simulink model "newsldrt2018"  (R2018b)
settings: Solver=ode5  StartTime=0.0  StopTime=10  FixedStep=1  RelTol=1e-3  EnableMultiTasking=on
model workspace (MAT data in the model file):
  A = 20
  a = 2
  b = 5
libraries: simulink x1
settings Model: Creator=The MathWorks, Inc.  LastModifiedBy=hp
settings SolverCC: ConcurrentTasks=on  PositivePriorityOrder=on
settings DataIOCC: ExternalInput=getinputstruct(op_watertank_comp_design)  InitialState=getstatestruct(op_watertank_comp_design)  LimitDataPoints=on  SaveFormat=Array  SignalLoggingName=logsOut
settings OptimizationCC: BlockReduction=off  OptimizeBlockIOStorage=off  ExpressionDepthLimit=2147483647  InitFltsAndDblsToZero=on  EfficientMapNaN2IntZero=off
settings DebuggingCC: AlgebraicLoopMsg=none  SaveWithParameterizedLinksMsg=none  UnderspecifiedInitializationDetection=Classic  MergeDetectMultiDrivingBlocksExec=none  SignalResolutionControl=TryResolveAllWithWarning  FcnCallInpInsideContextMsg=warning  UnconnectedInputMsg=none  UnconnectedOutputMsg=none  UnconnectedLineMsg=none  AllowSymbolicDim=off  StateNameClashWarn=warning  SFUnexpectedBacktrackingDiag=warning  SFNoUnconditionalDefaultTransitionDiag=warning  SFExecutionAtInitializationDiag=none
settings ModelReferenceCC: PropagateSignalLabelsOutOfModel=off
settings SFSimCC: SimUseLocalCustomCode=off
settings RTWCC: Description=Simulink Desktop Real-Time  SystemTargetFile=sldrt.tlc  TemplateMakefile=sldrt.tmf  RTWUseLocalCustomCode=off  Toolchain=Simulink Real-Time Toolchain  BuildConfiguration=Faster Runs  TargetLang=C++  RTWCompilerOptimization=on
settings CodeAppCC: MaxIdLength=95  StateflowObjectComments=on
settings SimulinkDesktopRealTimeCC: TargetPreCompLibLocation=D:\matlab\toolbox\sldrt\lib\win64  TargetLangStandard=C++03 (ISO)  ExtModeMexArgs=1
settings ConfigComp: CovMetricSettings=dw  CovSaveCumulativeToWorkspaceVar=on  CovSaveSingleToWorkspaceVar=on  CovExternalEMLEnable=off  CovSFcnEnable=off

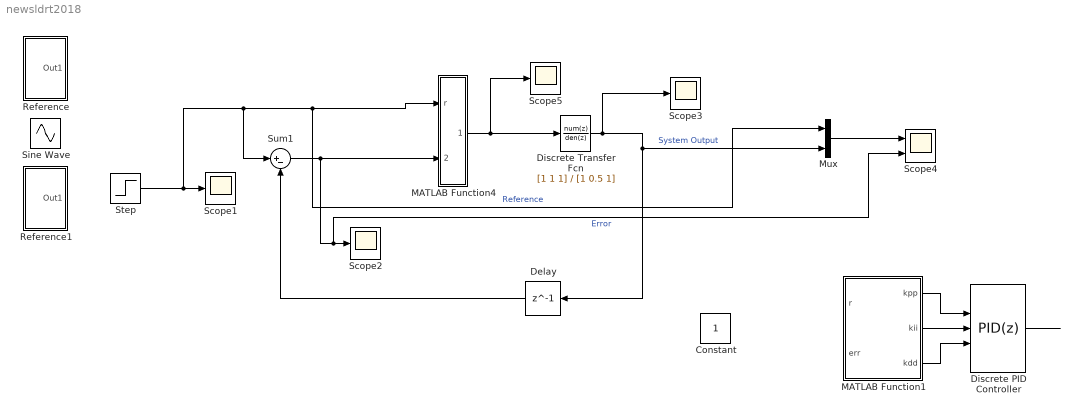
== system newsldrt2018 ==
  Constant : Constant
  Delay : Delay  DelayLength=1
  Discrete Transfer Fcn : DiscreteTransferFcn  Numerator=[1 1 1]  Denominator=[1 0.5 1]  SampleTime=0.002
  Discrete PID Controller : simulink/Continuous/PID Controller  Controller=PID  Form=Parallel  TimeDomain=Discrete-time  SampleTime=0.002  IntegratorMethod=Forward Euler  ControllerParametersSource=external  P=1  I=1  D=0  UseFilter=on  N=100  TunerSelectOption=Transfer Function Based (PID Tuner App)  InitialConditionSource=internal  InitialConditionForIntegrator=0  InitialConditionForFilter=0  DifferentiatorICPrevScaledInput=0  ExternalReset=none  TrackingMode=off  Kt=1  LimitOutput=on  UpperSaturationLimit=10  LowerSaturationLimit=0  LinearizeAsGain=off  AntiWindupMode=back-calculation  Kb=1  POutMin=[]  POutMax=[]  IOutMin=[]  IOutMax=[]  DOutMin=[]  DOutMax=[]  NOutMin=[]  NOutMax=[]  SumOutMin=[]  SumOutMax=[]  SaturationOutMin=[]  SaturationOutMax=[]  PParamMin=[]  PParamMax=[]  IParamMin=[]  IParamMax=[]  DParamMin=[]  DParamMax=[]  NParamMin=[]  NParamMax=[]  KbParamMin=[]  KbParamMax=[]  KtParamMin=[]  KtParamMax=[]  KbOutMin=[]  KbOutMax=[]  KtOutMin=[]  KtOutMax=[]  IntegratorOutMin=[]  IntegratorOutMax=[]  FilterOutMin=[]  FilterOutMax=[]  SumI1OutMin=[]  SumI1OutMax=[]  SumI2OutMin=[]  SumI2OutMax=[]  SumI3OutMin=[]  SumI3OutMax=[]  SumI4OutMin=[]  SumI4OutMax=[]  SumDOutMin=[]  SumDOutMax=[]  DifferentiatorOutMin=[]  DifferentiatorOutMax=[]  FilterDiffOutCoefMin=[]  FilterDiffOutCoefMax=[]  ReciprocalOutMin=[]  ReciprocalOutMax=[]  SumDenOutMin=[]  SumDenOutMax=[]  SumNumOutMin=[]  SumNumOutMax=[]  DivideOutMin=[]  DivideOutMax=[]  IntegratorContinuousStateAttributes=''  IntegratorStateMustResolveToSignalObject=off  IntegratorRTWStateStorageClass=Auto  FilterContinuousStateAttributes=''  FilterStateMustResolveToSignalObject=off  FilterRTWStateStorageClass=Auto  ParallelPVariant=ExternalParameters  IdealPVariant=Disabled  IVariant=ExternalParameters  DVariant=ExternalParameters  IntegratorVariant=Discrete  SatVariant=Enabled  AWVariant=BackCalculation  PCopyVariant=Disabled  TRVariant=Disabled  FdbkBlocksVariant=Forward  IdealPFdbkVariant=Disabled  SatFdbkVariant=Disabled  DerivativeFilterVariant=ForwardEulerFilter  NVariant=ExternalParameters  NCopyVariant=Disabled  FilterICVariant=InternalICsFilter  IntegratorICVariant=InternalICs  ExternalResetVariant=Disabled  TRSumVariant=Passthrough  SumFdbkVariant=Disabled  SumVariant=Sum_PID
  MATLAB Function1 : MATLAB Function  TreatAsAtomicUnit=on
  MATLAB Function4 : MATLAB Function  TreatAsAtomicUnit=on
  Mux : Mux  Inputs=2
  Reference : Subsystem
  Reference1 : Subsystem
  Scope{1..3,5} (4 alike) : Scope
  Scope4 : Scope  NumInputPorts=2
  Sine Wave : Sin  Bias=1  SampleTime=0.002
  Step : Step  Before=1  SampleTime=0.002
  Sum1 : Sum  Inputs=|+-  SaturateOnIntegerOverflow=on
  wires:
  Sum1/1 -> MATLAB Function4/2(err), Scope4/2, Scope2/1  "Error"
  Discrete Transfer Fcn/1 -> Delay/1, Mux/2, Scope3/1  "System Output"
  Step/1 -> MATLAB Function4/1(r), Mux/1, Sum1/1, Scope1/1  "Reference"
  Mux/1 -> Scope4/1
  Delay/1 -> Sum1/2
  MATLAB Function1/2(kii) -> Discrete PID Controller/3
  Discrete PID Controller/1 -> ?
  ? -> Discrete PID Controller/5
  MATLAB Function1/3(kdd) -> Discrete PID Controller/4
  ? -> Discrete PID Controller/1  "Error"
  MATLAB Function1/1(kpp) -> Discrete PID Controller/2
  MATLAB Function4/1(control) -> Scope5/1, Discrete Transfer Fcn/1

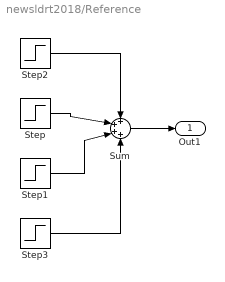
== system newsldrt2018/Reference ==
  Step : Step  Time=5  After=2  SampleTime=0.002
  Step1 : Step  Time=7  After=-3  SampleTime=0.002
  Step2 : Step  Time=3  Before=1  After=2  SampleTime=0.002
  Step3 : Step  Time=9  SampleTime=0.002
  Sum : Sum  Inputs=++++
  Out1 : Outport
  wires:
  Step1/1 -> Sum/3
  Sum/1 -> Out1/1
  Step/1 -> Sum/2
  Step2/1 -> Sum/1
  Step3/1 -> Sum/4

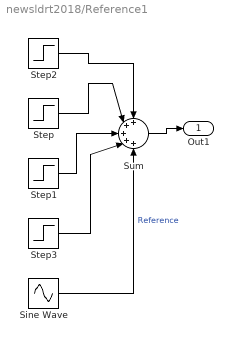
== system newsldrt2018/Reference1 ==
  Sine Wave : Sin  Bias=1  SampleTime=0
  Step : Step  Time=5  After=2  SampleTime=0
  Step1 : Step  Time=7  After=-3  SampleTime=0
  Step2 : Step  Time=3  Before=1  After=2  SampleTime=0
  Step3 : Step  Time=9  SampleTime=0
  Sum : Sum  Inputs=+++++
  Out1 : Outport
  wires:
  Step3/1 -> Sum/4
  Step2/1 -> Sum/1
  Step/1 -> Sum/2
  Sum/1 -> Out1/1
  Step1/1 -> Sum/3
  Sine Wave/1 -> Sum/5  "Reference"

== matlab function newsldrt2018/MATLAB Function1 ==
  settings: updateMethod=DISCRETE  sampleTime=0.002
  data: r input; kpp output; err input; kii output; kdd output
function [kpp,kii,kdd]  = fcn(r,err)
persistent Wij_c_p W1j_c_p S_prev_c_p e_prev_c_p u_prev_c_p u_prev_e_P control_prev
        if isempty(Wij_c_p)
        Wij_c_p = 0.05*rand(4,4);
        end
        if isempty(W1j_c_p)
        W1j_c_p = 0.05*rand(1,4);
        end
        if isempty(S_prev_c_p)
        S_prev_c_p = [0.1 0.2 0.3 0.4];
        end
        if isempty(e_prev_c_p)
        e_prev_c_p = 1;
        end
        if isempty(err)
        err = 1;
        end
        if isempty(u_prev_c_p)
        u_prev_c_p = 0;
        end
        if isempty(u_prev_e_P)
        u_prev_e_P = 0.05;
        end
        if isempty(control_prev)
        control_prev = 0;
        end
       % ********
           persistent e e_prev1 e_prev2 e_prev3 error_status
       error_status = 1;
       while true
            if isempty(e)
                e = err
                e_prev1 = 1
                e_prev2 = 1
                e_prev3 = 1
                error_status = 2;
                break
            elseif error_status == 2
                e_prev1 = e
                e = err
                e_prev2
                e_prev3
                error_status = 3
                break
            elseif error_status == 3
                e_prev2 = e_prev1
                e_prev1  = e
                e = err
                e_prev3
                error_status == 4
                break
            elseif error_status == 4
                e_prev3 =e_prev2
                e_prev2 = e_prev1
                e_prev1 = e
                e = err
                error_status == 5
                break
            else
                e_prev3 =e_prev2
                e_prev2 = e_prev1
                e_prev1 = e
                e = err
                break
            end
       end
       %***********
       persistent xp xp_prev1 xp_prev2 xp_prev3 xp_status
       xp_status = 1;
       while true
            if isempty(xp)
                xp = r
                xp_prev1 = 1
                xp_prev2 = 1
                xp_prev3 = 1
                xp_status = 2;
                break
            elseif xp_status == 2
                xp_prev1 = xp
                xp = r
                xp_prev2
                xp_prev3
                xp_status = 3
                break
            elseif xp_status == 3
                xp_prev2 = xp_prev1
                xp_prev1  = xp
                xp = r
                xp_prev3
                xp_status == 4
                break
            elseif xp_status == 4
                xp_prev3 =xp_prev2
                xp_prev2 = xp_prev1
                xp_prev1 = xp
                xp = r
                xp_status == 5
                break
            else
                xp_prev3 =xp_prev2
                xp_prev2 = xp_prev1
                xp_prev1 = xp
                xp = r
                break
            end
       end
       %******
       persistent Kp Ki Kd Kp_prev Ki_prev Kd_prev
        if isempty(Kp)
        Kp = 0.0432;
        end
        if isempty(Ki)
        Ki = 0.2007;
        end
        if isempty(Kd)
        Kd = 0.0043;
        end
        if isempty(Kp_prev)
        Kp_prev = 0;
        end
        if isempty(Ki_prev)
        Ki_prev = 0;
        end
        if isempty(Kd_prev)
        Kd_prev = 0;
        end
%  control = control_prev + Kp*(e_prev1 - e_prev2) + Ki*e_prev1 + Kd*(e_prev1 - 2*e_prev2 + e_prev3);
%  control_prev = control;
% input layer
net1_c_p = [xp;xp_prev1;xp_prev2;xp_prev3];
O1_c_p = net1_c_p;

% hidden layyer 
S_c_p = zeros (1,4);
 for j = 1:4
       S_c_p(j) = tanh(Wij_c_p(j,1)*xp+Wij_c_p(j,2)*xp_prev1 + Wij_c_p(j,3)*xp_prev2 + Wij_c_p(j,4)*xp_prev3);
 end
O2_c_p = zeros(1,4);
O2_c_p = [S_c_p(1),S_c_p(2),S_c_p(3),S_c_p(4)];

%output layer
net3_c_p = 0;
net3_c_p = W1j_c_p.*O2_c_p;
u_c_p = 0.5*(1+tanh(net3_c_p(1,1)+ net3_c_p(1,2) + net3_c_p(1,3)+net3_c_p(1,4)));

%% updating weights
B_c_p = 0.025;
d_c_p = u_prev_e_P;
sigma_c_p = sqrt(B_c_p)*e_prev1 + d_c_p;

%W1j updating
for j = 1 :4
    W1j_c_p(j) = sigma_c_p/(4*(S_prev_c_p(j))); %changed it to mean spc
end

%Wij updating
for j = 1:4
    Wij_c_p(j,1) = (1/(4*xp))*atanh(sigma_c_p/(4*W1j_c_p(1,j))); % Not OK
end
for j = 1:4
    Wij_c_p(j,2) = (1/(4*xp_prev1))*atanh(sigma_c_p/(4*W1j_c_p(1,j))); % Not OK
end
for j = 1:4
    Wij_c_p(j,3) = (1/(4*xp_prev2))*atanh(sigma_c_p/(4*W1j_c_p(1,j))); % Not OK
end
for j = 1:4
    Wij_c_p(j,4) = (1/(4*xp_prev3))*atanh(sigma_c_p/(4*W1j_c_p(1,j))); % Not OK
end

%% NNE
persistent Wij_e_p W1j_e_p S_prev_e_p e_prev_e_p  
        if isempty(Wij_e_p)
        Wij_e_p = 0.05*rand(4,4);
        end
        if isempty(W1j_e_p)
        W1j_e_p = 0.05*rand(1,4);
        end
        if isempty(S_prev_e_p)
        S_prev_e_p = [0.1 0.2 0.3 0.4];
        end
        if isempty(e_prev_e_p)
        e_prev_e_p = 1;
        end
    
% input layer
net1_e_p = [xp;xp_prev1;xp_prev2;xp_prev3];
O1_e_p = net1_e_p;

% hidden layyer 
S_e_p = zeros (1,4);
 for j = 1:4
       S_e_p(j) = tanh(Wij_e_p(j,1)*xp+Wij_e_p(j,2)*xp_prev1 + Wij_e_p(j,3)*xp_prev2 + Wij_e_p(j,4)*xp_prev3);
 end
O2_e_p = zeros(1,4);
O2_e_p = [S_e_p(1),S_e_p(2),S_e_p(3),S_e_p(4)];

%output layer
net3_e_p = 0;
net3_e_p = W1j_e_p.*O2_e_p;
u_e_p = 0.5*(1+tanh(net3_e_p(1,1)+ net3_e_p(1,2) + net3_e_p(1,3)+net3_e_p(1,4)));

%% updating weights
e_e_p = u_e_p - u_c_p;
B_e_p = 0.025;
d_e_p = u_c_p;
sigma_e_p = sqrt(B_e_p)*e_prev_e_p + d_e_p;
for j = 1 :4
    W1j_e_p(j) = sigma_e_p/(4*(S_prev_e_p(j))); %changed it to mean spc
end

for j = 1:4
    Wij_e_p(j,1) = (1/(4*xp))*atanh(sigma_e_p/(4*W1j_e_p(1,j))); % Not OK
end
for j = 1:4
    Wij_e_p(j,2) = (1/(4*xp_prev1))*atanh(sigma_e_p/(4*W1j_e_p(1,j))); % Not OK
end
for j = 1:4
    Wij_e_p(j,3) = (1/(4*xp_prev2))*atanh(sigma_e_p/(4*W1j_e_p(1,j))); % Not OK
end
for j = 1:4
    Wij_e_p(j,4) = (1/(4*xp_prev3))*atanh(sigma_e_p/(4*W1j_e_p(1,j))); % Not OK
end

%**************
S_prev_c_p = S_c_p;
e_prev_c_p = err;
S_prev_e_p = S_e_p;
e_prev_e_p = e_e_p;
u_prev_e_P = u_e_p;

%% NNI
persistent Wij_c_i W1j_c_i S_prev_c_i e_prev_c_i u_prev_c_i u_prev_e_i error_integral
    if isempty(Wij_c_i)
        Wij_c_i = 0.05*rand(4,4);
    end
    if isempty(W1j_c_i)
        W1j_c_i = 0.05*rand(1,4);
    end
        if isempty(S_prev_c_i)
        S_prev_c_i = [0.1 0.2 0.3 0.4];
        end
        if isempty(e_prev_c_i)
        e_prev_c_i = 1;
        end
        if isempty(err)
        err = 1;
        end
        if isempty(u_prev_c_i)
        u_prev_c_i = 0;
        end
        if isempty(u_prev_e_i)
        u_prev_e_i = 0.05;
        end
        if isempty(error_integral)
        error_integral = 1;
        end

    
% input layer
net1_c_i = [xp;xp_prev1;xp_prev2;xp_prev3];
O1_c_i = net1_c_i;

% hidden layyer 
S_c_i = zeros (1,4);
 for j = 1:4
       S_c_i(j) = tanh(Wij_c_i(j,1)*xp+Wij_c_i(j,2)*xp_prev1 + Wij_c_i(j,3)*xp_prev2 + Wij_c_i(j,4)*xp_prev3);
 end
O2_c_i = zeros(1,4);
O2_c_i = [S_c_i(1),S_c_i(2),S_c_i(3),S_c_i(4)]; 
%output layer
net3_c_i = 0;
net3_c_i = W1j_c_i.*O2_c_i;
u_c_i = 0.5*(1+tanh(net3_c_i(1,1)+ net3_c_i(1,2) + net3_c_i(1,3)+net3_c_i(1,4)));

%% updating weights
B_c_i = 0.025;
d_c_i = u_prev_e_i;
sigma_c_i = sqrt(B_c_i)*error_integral + d_c_i;
error_integral = e + error_integral;
for j = 1 :4
    W1j_c_i(j) = sigma_c_i/(4*(S_prev_c_i(j))); %changed it to mean spc
end

for j = 1:4
    Wij_c_i(j,1) = (1/(4*xp))*atanh(sigma_c_i/(4*W1j_c_i(1,j))); % Not OK
end
for j = 1:4
    Wij_c_i(j,2) = (1/(4*xp_prev1))*atanh(sigma_c_i/(4*W1j_c_i(1,j))); % Not OK
end
for j = 1:4
    Wij_c_i(j,3) = (1/(4*xp_prev2))*atanh(sigma_c_i/(4*W1j_c_i(1,j))); % Not OK
end
for j = 1:4
    Wij_c_i(j,4) = (1/(4*xp_prev3))*atanh(sigma_c_i/(4*W1j_c_i(1,j))); % Not OK
end

%% NNE
persistent Wij_e_i W1j_e_i S_prev_e_i e_prev_e_i  
    if isempty(Wij_e_i)
        Wij_e_i = 0.05*rand(4,4);
    end
    if isempty(W1j_e_i)
        W1j_e_i = 0.05*rand(1,4);
    end
        if isempty(S_prev_e_i)
        S_prev_e_i = [0.1 0.2 0.3 0.4];
        end
        if isempty(e_prev_e_i)
        e_prev_e_i = 1;
        end
    
% input layer
net1_e_i = [xp;xp_prev1;xp_prev2;xp_prev3];
O1_e_i = net1_e_i;
% hidden layyer 
S_e_i = zeros (1,4);
 for j = 1:4
       S_e_i(j) = tanh(Wij_e_i(j,1)*xp+Wij_e_i(j,2)*xp_prev1 + Wij_e_i(j,3)*xp_prev2 + Wij_e_i(j,4)*xp_prev3);
 end
O2_e_i = zeros(1,4);
O2_e_i = [S_e_i(1),S_e_i(2),S_e_i(3),S_e_i(4)]; 
%output layer
net3_e_i = 0;
net3_e_i = W1j_e_i.*O2_e_i;
u_e_i = 0.5*(1+tanh(net3_e_i(1,1)+ net3_e_i(1,2) + net3_e_i(1,3)+net3_e_i(1,4)));

%% updating weights
e_e_i = u_e_i - u_c_i;
B_e_i = 0.025;
d_e_i = u_c_i;
sigma_e_i = sqrt(B_e_i)*e_prev_e_i + d_e_i;
for j = 1 :4
    W1j_e_i(j) = sigma_e_i/(4*(S_prev_e_i(j))); %changed it to mean spc
end

for j = 1:4
    Wij_e_i(j,1) = (1/(4*xp))*atanh(sigma_e_i/(4*W1j_e_i(1,j))); % Not OK
end
for j = 1:4
    Wij_e_i(j,2) = (1/(4*xp_prev1))*atanh(sigma_e_i/(4*W1j_e_i(1,j))); % Not OK
end
for j = 1:4
    Wij_e_i(j,3) = (1/(4*xp_prev2))*atanh(sigma_e_i/(4*W1j_e_i(1,j))); % Not OK
end
for j = 1:4
    Wij_e_i(j,4) = (1/(4*xp_prev3))*atanh(sigma_e_i/(4*W1j_e_i(1,j))); % Not OK
end

%**************
S_prev_c_i = S_c_i;
e_prev_c_i = err;
S_prev_e_i = S_e_i;
e_prev_e_i = e_e_i;
u_prev_e_i = u_e_i;

%% NND
persistent Wij_c_d W1j_c_d S_prev_c_d e_prev_c_d u_prev_c_d u_prev_e_d error_derivative
    if isempty(Wij_c_d)
        Wij_c_d = 0.05*rand(4,4);
    end
    if isempty(W1j_c_d)
        W1j_c_d = 0.05*rand(1,4);
    end
        if isempty(S_prev_c_d)
        S_prev_c_d = [0.1 0.2 0.3 0.4];
        end
        if isempty(e_prev_c_d)
        e_prev_c_d = 1;
        end
        if isempty(u_prev_c_d)
        u_prev_c_d = 0;
        end
        if isempty(u_prev_e_d)
        u_prev_e_d = 0.05;
        end
        if isempty(error_derivative)
        error_derivative = 1;
        end

   
% input layer
net1_c_d = [xp;xp_prev1;xp_prev2;xp_prev3];
O1_c_d = net1_c_d;
% hidden layyer 
S_c_d = zeros (1,4);
 for j = 1:4
       S_c_d(j) = tanh(Wij_c_d(j,1)*xp+Wij_c_d(j,2)*xp_prev1 + Wij_c_d(j,3)*xp_prev2 + Wij_c_d(j,4)*xp_prev3);
 end

O2_c_d = zeros(1,4);
O2_c_d = [S_c_d(1),S_c_d(2),S_c_d(3),S_c_d(4)]; 
%output layer
net3_c_d = 0;
net3_c_d = W1j_c_d.*O2_c_d;
u_c_d = 0.5*(1+tanh(net3_c_d(1,1)+ net3_c_d(1,2) + net3_c_d(1,3)+net3_c_d(1,4)));

%% updating weights
B_c_d = 0.025;
d_c_d = u_prev_e_d;

sigma_c_d = sqrt(B_c_d)*error_derivative + d_c_d;
 error_derivative = (e - e_prev1)/0.002; %need to be fixed
for j = 1 :4
    W1j_c_d(j) = sigma_c_d/(4*(S_prev_c_d(j))); %changed it to mean spc
end
% W1j = sigma / (4*S_prev);

for j = 1:4
    Wij_c_d(j,1) = (1/(4*xp))*atanh(sigma_c_d/(4*W1j_c_d(1,j))); % Not OK
end
for j = 1:4
    Wij_c_d(j,2) = (1/(4*xp_prev1))*atanh(sigma_c_d/(4*W1j_c_d(1,j))); % Not OK
end
for j = 1:4
    Wij_c_d(j,3) = (1/(4*xp_prev2))*atanh(sigma_c_d/(4*W1j_c_d(1,j))); % Not OK
end
for j = 1:4
    Wij_c_d(j,4) = (1/(4*xp_prev3))*atanh(sigma_c_d/(4*W1j_c_d(1,j))); % Not OK
end
%% NNE
persistent Wij_e_d W1j_e_d S_prev_e_d e_prev_e_d  
    if isempty(Wij_e_d)
        Wij_e_d = 0.05*rand(4,4);
    end
    if isempty(W1j_e_d)
        W1j_e_d = 0.05*rand(1,4);
    end
        if isempty(S_prev_e_d)
        S_prev_e_d = [0.1 0.2 0.3 0.4];
        end
        if isempty(e_prev_e_d)
        e_prev_e_d = 1;
        end
    
% input layer
net1_e_d = [xp;xp_prev1;xp_prev2;xp_prev3];
O1_e_d = net1_e_d;
% hidden layyer 
S_e_d = zeros (1,4);
 for j = 1:4
       S_e_d(j) = tanh(Wij_e_d(j,1)*xp+Wij_e_d(j,2)*xp_prev1 + Wij_e_d(j,3)*xp_prev2 + Wij_e_d(j,4)*xp_prev3);
 end
O2_e_d = zeros(1,4);
O2_e_d = [S_e_d(1),S_e_d(2),S_e_d(3),S_e_d(4)]; 
%output layer
net3_e_d = 0;
net3_e_d = W1j_e_d.*O2_e_d;
u_e_d = 0.5*(1+tanh(net3_e_d(1,1)+ net3_e_d(1,2) + net3_e_d(1,3)+net3_e_d(1,4)));
%% updating weights
e_e_d = u_e_d - u_c_d;
B_e_d = 0.8;
d_e_d = u_c_d;
sigma_e_d = sqrt(B_e_d)*e_prev_e_d + d_e_d;
for j = 1 :4
    W1j_e_d(j) = sigma_e_d/(4*(S_prev_e_d(j))); %changed it to mean spc
end

for j = 1:4
    Wij_e_d(j,1) = (1/(4*xp))*atanh(sigma_e_d/(4*W1j_e_d(1,j))); % Not OK
end
for j = 1:4
    Wij_e_d(j,2) = (1/(4*xp_prev1))*atanh(sigma_e_d/(4*W1j_e_d(1,j))); % Not OK
end
for j = 1:4
    Wij_e_d(j,3) = (1/(4*xp_prev2))*atanh(sigma_e_d/(4*W1j_e_d(1,j))); % Not OK
end
for j = 1:4
    Wij_e_d(j,4) = (1/(4*xp_prev3))*atanh(sigma_e_d/(4*W1j_e_d(1,j))); % Not OK
end

% Kp = u_c_p/3.33;
% Ki = u_c_i/3.33;
% Kd = u_c_d/20;
% Kp_prev = Kp;
% Ki_prev = Ki;
% Kd_prev = Kd;
% % if e > 1e-5
Kp = u_c_p/3.33;
Ki = u_c_i/3.33;
Kd = u_c_d/20;
Kp_prev = Kp;
Ki_prev = Ki;
Kd_prev = Kd;
kpp = Kp;
kii = Ki;
kdd = Kd;
% % else
% %     Kp = Kp_prev;
% %     Ki = Ki_prev;
% %     Kd = Kd_prev;
% % end
%  control = control_prev + Kp*(e_prev1 - e_prev2) + Ki*e_prev1 + Kd*(e_prev1 - 2*e_prev2 + e_prev3);
%  control_prev = control;
%**************
S_prev_c_d = S_c_d;
e_prev_c_d = err;
S_prev_e_d = S_e_d;
e_prev_e_d = e_e_d;
u_prev_e_d = u_e_d;

== matlab function newsldrt2018/MATLAB Function4 ==
  settings: updateMethod=DISCRETE  sampleTime=0.002
  data: r input; control output; err input
function control  = fcn(r,err)
persistent Wij_c_p W1j_c_p S_prev_c_p e_prev_c_p u_prev_c_p u_prev_e_P control_prev
        if isempty(Wij_c_p)
        Wij_c_p = 0.05*rand(4,4);
        end
        if isempty(W1j_c_p)
        W1j_c_p = 0.05*rand(1,4);
        end
        if isempty(S_prev_c_p)
        S_prev_c_p = [0.1 0.2 0.3 0.4];
        end
        if isempty(e_prev_c_p)
        e_prev_c_p = 1;
        end
        if isempty(err)
        err = 1;
        end
        if isempty(u_prev_c_p)
        u_prev_c_p = 0;
        end
        if isempty(u_prev_e_P)
        u_prev_e_P = 0.05;
        end
        if isempty(control_prev)
        control_prev = 0;
        end
       % ********
           persistent e e_prev1 e_prev2 e_prev3 error_status
       error_status = 1;
       while true
            if isempty(e)
                e = err
                e_prev1 = 1
                e_prev2 = 1
                e_prev3 = 1
                error_status = 2;
                break
            elseif error_status == 2
                e_prev1 = e
                e = err
                e_prev2
                e_prev3
                error_status = 3
                break
            elseif error_status == 3
                e_prev2 = e_prev1
                e_prev1  = e
                e = err
                e_prev3
                error_status == 4
                break
            elseif error_status == 4
                e_prev3 =e_prev2
                e_prev2 = e_prev1
                e_prev1 = e
                e = err
                error_status == 5
                break
            else
                e_prev3 =e_prev2
                e_prev2 = e_prev1
                e_prev1 = e
                e = err
                break
            end
       end
       %***********
       persistent xp xp_prev1 xp_prev2 xp_prev3 xp_status
       xp_status = 1;
       while true
            if isempty(xp)
                xp = r
                xp_prev1 = 1
                xp_prev2 = 1
                xp_prev3 = 1
                xp_status = 2;
                break
            elseif xp_status == 2
                xp_prev1 = xp
                xp = r
                xp_prev2
                xp_prev3
                xp_status = 3
                break
            elseif xp_status == 3
                xp_prev2 = xp_prev1
                xp_prev1  = xp
                xp = r
                xp_prev3
                xp_status == 4
                break
            elseif xp_status == 4
                xp_prev3 =xp_prev2
                xp_prev2 = xp_prev1
                xp_prev1 = xp
                xp = r
                xp_status == 5
                break
            else
                xp_prev3 =xp_prev2
                xp_prev2 = xp_prev1
                xp_prev1 = xp
                xp = r
                break
            end
       end
       %******
       persistent Kp Ki Kd Kp_prev Ki_prev Kd_prev
        if isempty(Kp)
        Kp = 0.0432;
        end
        if isempty(Ki)
        Ki = 0.2007;
        end
        if isempty(Kd)
        Kd = 0.0043;
        end
        if isempty(Kp_prev)
        Kp_prev = 0;
        end
        if isempty(Ki_prev)
        Ki_prev = 0;
        end
        if isempty(Kd_prev)
        Kd_prev = 0;
        end
%  control = control_prev + Kp*(e_prev1 - e_prev2) + Ki*e_prev1 + Kd*(e_prev1 - 2*e_prev2 + e_prev3);
%  control_prev = control;
% input layer
net1_c_p = [xp;xp_prev1;xp_prev2;xp_prev3];
O1_c_p = net1_c_p;

% hidden layyer 
S_c_p = zeros (1,4);
 for j = 1:4
       S_c_p(j) = tanh(Wij_c_p(j,1)*xp+Wij_c_p(j,2)*xp_prev1 + Wij_c_p(j,3)*xp_prev2 + Wij_c_p(j,4)*xp_prev3);
 end
O2_c_p = zeros(1,4);
O2_c_p = [S_c_p(1),S_c_p(2),S_c_p(3),S_c_p(4)];

%output layer
net3_c_p = 0;
net3_c_p = W1j_c_p.*O2_c_p;
u_c_p = 0.5*(1+tanh(net3_c_p(1,1)+ net3_c_p(1,2) + net3_c_p(1,3)+net3_c_p(1,4)));

%% updating weights
B_c_p = 0.025;
d_c_p = u_prev_e_P;
sigma_c_p = sqrt(B_c_p)*e_prev1 + d_c_p;

%W1j updating
for j = 1 :4
    W1j_c_p(j) = sigma_c_p/(4*(S_prev_c_p(j))); %changed it to mean spc
end

%Wij updating
for j = 1:4
    Wij_c_p(j,1) = (1/(4*xp))*atanh(sigma_c_p/(4*W1j_c_p(1,j))); % Not OK
end
for j = 1:4
    Wij_c_p(j,2) = (1/(4*xp_prev1))*atanh(sigma_c_p/(4*W1j_c_p(1,j))); % Not OK
end
for j = 1:4
    Wij_c_p(j,3) = (1/(4*xp_prev2))*atanh(sigma_c_p/(4*W1j_c_p(1,j))); % Not OK
end
for j = 1:4
    Wij_c_p(j,4) = (1/(4*xp_prev3))*atanh(sigma_c_p/(4*W1j_c_p(1,j))); % Not OK
end

%% NNE
persistent Wij_e_p W1j_e_p S_prev_e_p e_prev_e_p  
        if isempty(Wij_e_p)
        Wij_e_p = 0.05*rand(4,4);
        end
        if isempty(W1j_e_p)
        W1j_e_p = 0.05*rand(1,4);
        end
        if isempty(S_prev_e_p)
        S_prev_e_p = [0.1 0.2 0.3 0.4];
        end
        if isempty(e_prev_e_p)
        e_prev_e_p = 1;
        end
    
% input layer
net1_e_p = [xp;xp_prev1;xp_prev2;xp_prev3];
O1_e_p = net1_e_p;

% hidden layyer 
S_e_p = zeros (1,4);
 for j = 1:4
       S_e_p(j) = tanh(Wij_e_p(j,1)*xp+Wij_e_p(j,2)*xp_prev1 + Wij_e_p(j,3)*xp_prev2 + Wij_e_p(j,4)*xp_prev3);
 end
O2_e_p = zeros(1,4);
O2_e_p = [S_e_p(1),S_e_p(2),S_e_p(3),S_e_p(4)];

%output layer
net3_e_p = 0;
net3_e_p = W1j_e_p.*O2_e_p;
u_e_p = 0.5*(1+tanh(net3_e_p(1,1)+ net3_e_p(1,2) + net3_e_p(1,3)+net3_e_p(1,4)));

%% updating weights
e_e_p = u_e_p - u_c_p;
B_e_p = 0.025;
d_e_p = u_c_p;
sigma_e_p = sqrt(B_e_p)*e_prev_e_p + d_e_p;
for j = 1 :4
    W1j_e_p(j) = sigma_e_p/(4*(S_prev_e_p(j))); %changed it to mean spc
end

for j = 1:4
    Wij_e_p(j,1) = (1/(4*xp))*atanh(sigma_e_p/(4*W1j_e_p(1,j))); % Not OK
end
for j = 1:4
    Wij_e_p(j,2) = (1/(4*xp_prev1))*atanh(sigma_e_p/(4*W1j_e_p(1,j))); % Not OK
end
for j = 1:4
    Wij_e_p(j,3) = (1/(4*xp_prev2))*atanh(sigma_e_p/(4*W1j_e_p(1,j))); % Not OK
end
for j = 1:4
    Wij_e_p(j,4) = (1/(4*xp_prev3))*atanh(sigma_e_p/(4*W1j_e_p(1,j))); % Not OK
end

%**************
S_prev_c_p = S_c_p;
e_prev_c_p = err;
S_prev_e_p = S_e_p;
e_prev_e_p = e_e_p;
u_prev_e_P = u_e_p;

%% NNI
persistent Wij_c_i W1j_c_i S_prev_c_i e_prev_c_i u_prev_c_i u_prev_e_i error_integral
    if isempty(Wij_c_i)
        Wij_c_i = 0.05*rand(4,4);
    end
    if isempty(W1j_c_i)
        W1j_c_i = 0.05*rand(1,4);
    end
        if isempty(S_prev_c_i)
        S_prev_c_i = [0.1 0.2 0.3 0.4];
        end
        if isempty(e_prev_c_i)
        e_prev_c_i = 1;
        end
        if isempty(err)
        err = 1;
        end
        if isempty(u_prev_c_i)
        u_prev_c_i = 0;
        end
        if isempty(u_prev_e_i)
        u_prev_e_i = 0.05;
        end
        if isempty(error_integral)
        error_integral = 1;
        end

    
% input layer
net1_c_i = [xp;xp_prev1;xp_prev2;xp_prev3];
O1_c_i = net1_c_i;

% hidden layyer 
S_c_i = zeros (1,4);
 for j = 1:4
       S_c_i(j) = tanh(Wij_c_i(j,1)*xp+Wij_c_i(j,2)*xp_prev1 + Wij_c_i(j,3)*xp_prev2 + Wij_c_i(j,4)*xp_prev3);
 end
O2_c_i = zeros(1,4);
O2_c_i = [S_c_i(1),S_c_i(2),S_c_i(3),S_c_i(4)]; 
%output layer
net3_c_i = 0;
net3_c_i = W1j_c_i.*O2_c_i;
u_c_i = 0.5*(1+tanh(net3_c_i(1,1)+ net3_c_i(1,2) + net3_c_i(1,3)+net3_c_i(1,4)));

%% updating weights
B_c_i = 0.025;
d_c_i = u_prev_e_i;
sigma_c_i = sqrt(B_c_i)*error_integral + d_c_i;
error_integral = e + error_integral;
for j = 1 :4
    W1j_c_i(j) = sigma_c_i/(4*(S_prev_c_i(j))); %changed it to mean spc
end

for j = 1:4
    Wij_c_i(j,1) = (1/(4*xp))*atanh(sigma_c_i/(4*W1j_c_i(1,j))); % Not OK
end
for j = 1:4
    Wij_c_i(j,2) = (1/(4*xp_prev1))*atanh(sigma_c_i/(4*W1j_c_i(1,j))); % Not OK
end
for j = 1:4
    Wij_c_i(j,3) = (1/(4*xp_prev2))*atanh(sigma_c_i/(4*W1j_c_i(1,j))); % Not OK
end
for j = 1:4
    Wij_c_i(j,4) = (1/(4*xp_prev3))*atanh(sigma_c_i/(4*W1j_c_i(1,j))); % Not OK
end

%% NNE
persistent Wij_e_i W1j_e_i S_prev_e_i e_prev_e_i  
    if isempty(Wij_e_i)
        Wij_e_i = 0.05*rand(4,4);
    end
    if isempty(W1j_e_i)
        W1j_e_i = 0.05*rand(1,4);
    end
        if isempty(S_prev_e_i)
        S_prev_e_i = [0.1 0.2 0.3 0.4];
        end
        if isempty(e_prev_e_i)
        e_prev_e_i = 1;
        end
    
% input layer
net1_e_i = [xp;xp_prev1;xp_prev2;xp_prev3];
O1_e_i = net1_e_i;
% hidden layyer 
S_e_i = zeros (1,4);
 for j = 1:4
       S_e_i(j) = tanh(Wij_e_i(j,1)*xp+Wij_e_i(j,2)*xp_prev1 + Wij_e_i(j,3)*xp_prev2 + Wij_e_i(j,4)*xp_prev3);
 end
O2_e_i = zeros(1,4);
O2_e_i = [S_e_i(1),S_e_i(2),S_e_i(3),S_e_i(4)]; 
%output layer
net3_e_i = 0;
net3_e_i = W1j_e_i.*O2_e_i;
u_e_i = 0.5*(1+tanh(net3_e_i(1,1)+ net3_e_i(1,2) + net3_e_i(1,3)+net3_e_i(1,4)));

%% updating weights
e_e_i = u_e_i - u_c_i;
B_e_i = 0.025;
d_e_i = u_c_i;
sigma_e_i = sqrt(B_e_i)*e_prev_e_i + d_e_i;
for j = 1 :4
    W1j_e_i(j) = sigma_e_i/(4*(S_prev_e_i(j))); %changed it to mean spc
end

for j = 1:4
    Wij_e_i(j,1) = (1/(4*xp))*atanh(sigma_e_i/(4*W1j_e_i(1,j))); % Not OK
end
for j = 1:4
    Wij_e_i(j,2) = (1/(4*xp_prev1))*atanh(sigma_e_i/(4*W1j_e_i(1,j))); % Not OK
end
for j = 1:4
    Wij_e_i(j,3) = (1/(4*xp_prev2))*atanh(sigma_e_i/(4*W1j_e_i(1,j))); % Not OK
end
for j = 1:4
    Wij_e_i(j,4) = (1/(4*xp_prev3))*atanh(sigma_e_i/(4*W1j_e_i(1,j))); % Not OK
end

%**************
S_prev_c_i = S_c_i;
e_prev_c_i = err;
S_prev_e_i = S_e_i;
e_prev_e_i = e_e_i;
u_prev_e_i = u_e_i;

%% NND
persistent Wij_c_d W1j_c_d S_prev_c_d e_prev_c_d u_prev_c_d u_prev_e_d error_derivative
    if isempty(Wij_c_d)
        Wij_c_d = 0.05*rand(4,4);
    end
    if isempty(W1j_c_d)
        W1j_c_d = 0.05*rand(1,4);
    end
        if isempty(S_prev_c_d)
        S_prev_c_d = [0.1 0.2 0.3 0.4];
        end
        if isempty(e_prev_c_d)
        e_prev_c_d = 1;
        end
        if isempty(u_prev_c_d)
        u_prev_c_d = 0;
        end
        if isempty(u_prev_e_d)
        u_prev_e_d = 0.05;
        end
        if isempty(error_derivative)
        error_derivative = 1;
        end

   
% input layer
net1_c_d = [xp;xp_prev1;xp_prev2;xp_prev3];
O1_c_d = net1_c_d;
% hidden layyer 
S_c_d = zeros (1,4);
 for j = 1:4
       S_c_d(j) = tanh(Wij_c_d(j,1)*xp+Wij_c_d(j,2)*xp_prev1 + Wij_c_d(j,3)*xp_prev2 + Wij_c_d(j,4)*xp_prev3);
 end

O2_c_d = zeros(1,4);
O2_c_d = [S_c_d(1),S_c_d(2),S_c_d(3),S_c_d(4)]; 
%output layer
net3_c_d = 0;
net3_c_d = W1j_c_d.*O2_c_d;
u_c_d = 0.5*(1+tanh(net3_c_d(1,1)+ net3_c_d(1,2) + net3_c_d(1,3)+net3_c_d(1,4)));

%% updating weights
B_c_d = 0.025;
d_c_d = u_prev_e_d;

sigma_c_d = sqrt(B_c_d)*error_derivative + d_c_d;
 error_derivative = (e - e_prev1)/0.002; %need to be fixed
for j = 1 :4
    W1j_c_d(j) = sigma_c_d/(4*(S_prev_c_d(j))); %changed it to mean spc
end
% W1j = sigma / (4*S_prev);

for j = 1:4
    Wij_c_d(j,1) = (1/(4*xp))*atanh(sigma_c_d/(4*W1j_c_d(1,j))); % Not OK
end
for j = 1:4
    Wij_c_d(j,2) = (1/(4*xp_prev1))*atanh(sigma_c_d/(4*W1j_c_d(1,j))); % Not OK
end
for j = 1:4
    Wij_c_d(j,3) = (1/(4*xp_prev2))*atanh(sigma_c_d/(4*W1j_c_d(1,j))); % Not OK
end
for j = 1:4
    Wij_c_d(j,4) = (1/(4*xp_prev3))*atanh(sigma_c_d/(4*W1j_c_d(1,j))); % Not OK
end
%% NNE
persistent Wij_e_d W1j_e_d S_prev_e_d e_prev_e_d  
    if isempty(Wij_e_d)
        Wij_e_d = 0.05*rand(4,4);
    end
    if isempty(W1j_e_d)
        W1j_e_d = 0.05*rand(1,4);
    end
        if isempty(S_prev_e_d)
        S_prev_e_d = [0.1 0.2 0.3 0.4];
        end
        if isempty(e_prev_e_d)
        e_prev_e_d = 1;
        end
    
% input layer
net1_e_d = [xp;xp_prev1;xp_prev2;xp_prev3];
O1_e_d = net1_e_d;
% hidden layyer 
S_e_d = zeros (1,4);
 for j = 1:4
       S_e_d(j) = tanh(Wij_e_d(j,1)*xp+Wij_e_d(j,2)*xp_prev1 + Wij_e_d(j,3)*xp_prev2 + Wij_e_d(j,4)*xp_prev3);
 end
O2_e_d = zeros(1,4);
O2_e_d = [S_e_d(1),S_e_d(2),S_e_d(3),S_e_d(4)]; 
%output layer
net3_e_d = 0;
net3_e_d = W1j_e_d.*O2_e_d;
u_e_d = 0.5*(1+tanh(net3_e_d(1,1)+ net3_e_d(1,2) + net3_e_d(1,3)+net3_e_d(1,4)));
%% updating weights
e_e_d = u_e_d - u_c_d;
B_e_d = 0.8;
d_e_d = u_c_d;
sigma_e_d = sqrt(B_e_d)*e_prev_e_d + d_e_d;
for j = 1 :4
    W1j_e_d(j) = sigma_e_d/(4*(S_prev_e_d(j))); %changed it to mean spc
end

for j = 1:4
    Wij_e_d(j,1) = (1/(4*xp))*atanh(sigma_e_d/(4*W1j_e_d(1,j))); % Not OK
end
for j = 1:4
    Wij_e_d(j,2) = (1/(4*xp_prev1))*atanh(sigma_e_d/(4*W1j_e_d(1,j))); % Not OK
end
for j = 1:4
    Wij_e_d(j,3) = (1/(4*xp_prev2))*atanh(sigma_e_d/(4*W1j_e_d(1,j))); % Not OK
end
for j = 1:4
    Wij_e_d(j,4) = (1/(4*xp_prev3))*atanh(sigma_e_d/(4*W1j_e_d(1,j))); % Not OK
end

% Kp = u_c_p/3.33;
% Ki = u_c_i/3.33;
% Kd = u_c_d/20;
% Kp_prev = Kp;
% Ki_prev = Ki;
% Kd_prev = Kd;
% % if e > 1e-5
Kp = u_c_p/3.33;
Ki = u_c_i/3.33;
Kd = u_c_d/20;
Kp_prev = Kp;
Ki_prev = Ki;
Kd_prev = Kd;
% % else
% %     Kp = Kp_prev;
% %     Ki = Ki_prev;
% %     Kd = Kd_prev;
% % end
 control = control_prev + Kp*(e_prev1 - e_prev2) + Ki*e_prev1 + Kd*(e_prev1 - 2*e_prev2 + e_prev3);
 control_prev = control;
%**************
S_prev_c_d = S_c_d;
e_prev_c_d = err;
S_prev_e_d = S_e_d;
e_prev_e_d = e_e_d;
u_prev_e_d = u_e_d;
